simulink model "EXAM1_19b"  (Simulink 10.0)
settings: Solver=FixedStepAuto  StartTime=0.0  StopTime=20  FixedStep=0.01  RelTol=1e-3
settings Model: Creator=axs2437  LastModifiedBy=axs2437
settings DataIOCC: SaveFormat=Dataset  ReturnWorkspaceOutputs=on
settings OptimizationCC: LifeSpan=auto
settings DebuggingCC: UnderspecifiedInitializationDetection=Simplified  MergeDetectMultiDrivingBlocksExec=error  SFUnexpectedBacktrackingDiag=error  SFNoUnconditionalDefaultTransitionDiag=error  SFExecutionAtInitializationDiag=warning  ArithmeticOperatorsInVariantConditions=error
settings HardwareCC: ProdBitPerPointer=64  ProdBitPerSizeT=64  ProdBitPerPtrDiffT=64  ProdLargestAtomicFloat=Float  ProdIntDivRoundTo=Zero  ProdEndianess=LittleEndian  ProdWordSize=64  ProdHWDeviceType=Intel->x86-64 (Windows64)
settings ModelReferenceCC: PropagateSignalLabelsOutOfModel=on
settings SFSimCC: SimUseLocalCustomCode=on  CustomCodeUndefinedFunction=FilterOut
settings RTWCC: RTWUseLocalCustomCode=on
settings CodeAppCC: StateflowObjectComments=off
settings GRTTargetCC: TargetLangStandard=C99 (ISO)  CombineOutputUpdateFcns=on  GRTInterface=off
settings ConfigComp: CovMetricSettings=dwe  CovHtmlReporting=off  CovSaveCumulativeToWorkspaceVar=off  CovSaveSingleToWorkspaceVar=off

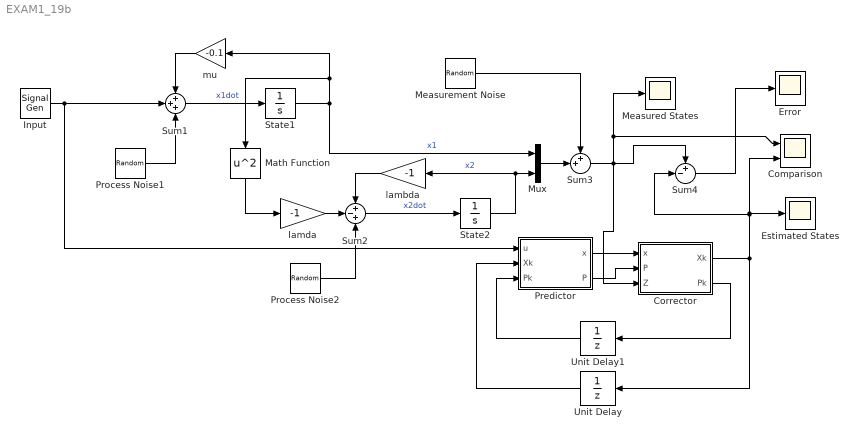
== system EXAM1_19b ==
  Comparison : Scope  NumInputPorts=2
  Corrector : MATLAB Function  TreatAsAtomicUnit=on
  Error : Scope
  Estimated States : Scope
  Input : SignalGenerator  WaveForm=square  Amplitude=3
  Math Function : Math  Operator=square  SignedPower=off  SaturateOnIntegerOverflow=on
  Measured States : Scope
  Measurement Noise : RandomNumber  Variance=[0.1 0.1]  Seed=[6 7]  SampleTime=0.01
  Mux : Mux  Inputs=2
  Predictor : MATLAB Function  TreatAsAtomicUnit=on
  Process Noise1 : RandomNumber  Seed=9  SampleTime=0.01
  Process Noise2 : RandomNumber  Seed=3  SampleTime=0.01
  State1 : Integrator  InitialCondition=5
  State2 : Integrator
  Sum1 : Sum  Inputs=+++
  Sum2 : Sum  Inputs=+-+
  Sum3 : Sum  Inputs=++|
  Sum4 : Sum  Inputs=+-|
  Unit Delay : UnitDelay  InitialCondition=[5 0]  SampleTime=-1  HasFrameUpgradeWarning=on
  Unit Delay1 : UnitDelay  InitialCondition=eye(2)*5  SampleTime=-1  HasFrameUpgradeWarning=on
  lambda : Gain  Gain=-1
  lamda : Gain  Gain=-1
  mu : Gain  Gain=-0.1
  wires:
  Predictor/1(x) -> Corrector/1(x)
  Predictor/2(P) -> Corrector/2(P)
  Corrector/1(Xk) -> Comparison/2, Estimated States/1, Sum4/2, Unit Delay/1
  Unit Delay/1 -> Predictor/2(Xk)
  Corrector/2(Pk) -> Unit Delay1/1
  Unit Delay1/1 -> Predictor/3(Pk)
  Sum1/1 -> State1/1  "x1dot"
  Sum2/1 -> State2/1  "x2dot"
  Input/1 -> Predictor/1(u), Sum1/2
  State1/1 -> Math Function/1, mu/1, Mux/1  "x1"
  mu/1 -> Sum1/1
  Process Noise1/1 -> Sum1/3
  State2/1 -> lambda/1, Mux/2  "x2"
  Process Noise2/1 -> Sum2/3
  lambda/1 -> Sum2/1
  lamda/1 -> Sum2/2
  Mux/1 -> Sum3/2
  Measurement Noise/1 -> Sum3/1
  Sum3/1 -> Sum4/1, Comparison/1, Measured States/1, Corrector/3(Z)
  Sum4/1 -> Error/1
  Math Function/1 -> lamda/1

== matlab function Corrector ==
  data: x input double; Xk output double; P input double; Pk output double; Z input double
function [Xk,Pk] = Corrector(x,P,Z)
H=eye(2); R=0.1*eye(2); Rd=R/0.01;
K=P*transpose(H)*inv(H*P*transpose(H)+Rd);
Pk=(eye(2)-K*H)*P*transpose(eye(2)-K*H)+K*Rd*transpose(K);
Xk=x+K*(Z-H*x);
end

== matlab function Predictor ==
  data: u input double; x output double size=2; Xk input double size=2; Pk input double; P output double
function [x,P] = Predictor(u,Xk,Pk)
mu=-0.1; lam=-1;
A = [mu 0;-2*lam*Xk(1) lam];
B= [1;0];
Ad=expm(A*0.01);
Bd=inv(A)*(Ad-eye(2))*B;
Q=eye(2);
F=[-A Q;zeros(2,2) transpose(A)];
G=expm(F*0.01);
Qd=transpose(G(3:4,3:4))*G(1:2,3:4); 
x=Ad*Xk + Bd*u;
P=(Ad*Pk*transpose(Ad)+Qd);
end
